simulink library "EmE_MBD_Blockset"  (R2018a)
settings: Solver=ode1  StartTime=0.0  StopTime=Inf  FixedStep=0.001  RelTol=1e-3  EnableMultiTasking=on
PostLoadFcn:
  | , if any(exist('dsrtsu_mdlpostloadfcn', 'file') == [2, 3, 6]), try dsrtsu_mdlpostloadfcn('Execute', bdroot); catch fprintf('Error in PostLoadFcn (dsrtsu_mdlpostloadfcn) for model "%s":\n %s\n', bdroot, lasterr); end, end,
undefined symbols (not defined in the file or in its folder): ENUM_TSC1_CONTROL_PURPOSE_T, gcbh, GLB_SWITCH_T
libraries: simulink x237, $bdroot x115, simulink_need_slupdate x26, MotoHawk_lib x13, simulink_extras x3
(part 6 of 11)

== system EmE_MBD_Blockset/User-Defined Functions/Snoop/CCP_ETC_SS2/Recieve Count ==
  Add : Sum  AccumDataTypeStr=uint8  OutDataTypeStr=uint8
  Constant : Constant  OutDataTypeStr=uint8
  Unit Delay : UnitDelay  SampleTime=-1
  motohawk_probe : MotoHawk_lib/Calibration & Probing Blocks/motohawk_probe  nam='CCP_Snoop_ETCrsp_cnt'  show_more=on  name_source=Use Parameter  read_level=1  view_as=Number  enum_struct={'Disabled', 'Enabled'}  vector_style=Wide Row  use_help_units=off  help=''  units=''  use_header_enum=off  row_header_enum={}  col_header_enum={}  use_min_max=off  min_val=-inf  max_val=inf  use_precision=off  precision=''  gain=1  offset=0  exp=1  use_mototune_group=on  mototune_group='CCP_Snoop'
      settings: SourceProductName=MotoHawk
  wires:
  Unit Delay/1 -> Add/2
  Add/1 -> Unit Delay/1, motohawk_probe/1
  Constant/1 -> Add/1

== system EmE_MBD_Blockset/User-Defined Functions/Snoop/Defaulting/DEFAULT1 ==
  signal : Inport
  reset_delay : Inport  Port=2
  f_defined : Inport  Port=3
  CCP_SIG_DEFAULT : Constant  Value=0
  FGND_RTI_ms : Constant  Value=10
  Switch : Switch  Criteria=u2 ~= 0
  Switch1 : Switch  Criteria=u2 ~= 0
  Turn_off_delay : $bdroot/Discrete/Turn_off_delay
  Unit Delay : UnitDelay  SampleTime=-1
  Signal : Outport
  F_Defined : Outport  Port=2
  wires:
  reset_delay/1 -> Turn_off_delay/2
  Turn_off_delay/1 -> Switch/2, F_Defined/1
  FGND_RTI_ms/1 -> Turn_off_delay/3
  Switch1/1 -> Switch/1, Unit Delay/1
  Unit Delay/1 -> Switch1/3
  Switch/1 -> Signal/1
  signal/1 -> Switch1/1
  CCP_SIG_DEFAULT/1 -> Switch/3
  f_defined/1 -> Turn_off_delay/1, Switch1/2

== system EmE_MBD_Blockset/User-Defined Functions/Snoop/Defaulting/DEFAULT10 ==
  signal : Inport
  reset_delay : Inport  Port=2
  f_defined : Inport  Port=3
  CCP_SIG_DEFAULT : Constant  Value=0
  FGND_RTI_ms : Constant  Value=10
  Switch : Switch  Criteria=u2 ~= 0
  Switch1 : Switch  Criteria=u2 ~= 0
  Turn_off_delay : $bdroot/Discrete/Turn_off_delay
  Unit Delay : UnitDelay  SampleTime=-1
  Signal : Outport
  F_Defined : Outport  Port=2
  wires:
  f_defined/1 -> Switch1/2, Turn_off_delay/1
  CCP_SIG_DEFAULT/1 -> Switch/3
  signal/1 -> Switch1/1
  Switch/1 -> Signal/1
  Unit Delay/1 -> Switch1/3
  Switch1/1 -> Unit Delay/1, Switch/1
  FGND_RTI_ms/1 -> Turn_off_delay/3
  Turn_off_delay/1 -> F_Defined/1, Switch/2
  reset_delay/1 -> Turn_off_delay/2

== system EmE_MBD_Blockset/User-Defined Functions/Snoop/Defaulting/DEFAULT11 ==
  signal : Inport
  reset_delay : Inport  Port=2
  f_defined : Inport  Port=3
  CCP_SIG_DEFAULT : Constant  Value=0
  FGND_RTI_ms : Constant  Value=10
  Switch : Switch  Criteria=u2 ~= 0
  Switch1 : Switch  Criteria=u2 ~= 0
  Turn_off_delay : $bdroot/Discrete/Turn_off_delay
  Unit Delay : UnitDelay  SampleTime=-1
  Signal : Outport
  F_Defined : Outport  Port=2
  wires:
  f_defined/1 -> Switch1/2, Turn_off_delay/1
  CCP_SIG_DEFAULT/1 -> Switch/3
  signal/1 -> Switch1/1
  Switch/1 -> Signal/1
  Unit Delay/1 -> Switch1/3
  Switch1/1 -> Unit Delay/1, Switch/1
  FGND_RTI_ms/1 -> Turn_off_delay/3
  Turn_off_delay/1 -> F_Defined/1, Switch/2
  reset_delay/1 -> Turn_off_delay/2

== system EmE_MBD_Blockset/User-Defined Functions/Snoop/Defaulting/DEFAULT12 ==
  signal : Inport
  reset_delay : Inport  Port=2
  f_defined : Inport  Port=3
  CCP_SIG_DEFAULT : Constant  Value=0
  FGND_RTI_ms : Constant  Value=10
  Switch : Switch  Criteria=u2 ~= 0
  Switch1 : Switch  Criteria=u2 ~= 0
  Turn_off_delay : $bdroot/Discrete/Turn_off_delay
  Unit Delay : UnitDelay  SampleTime=-1
  Signal : Outport
  F_Defined : Outport  Port=2
  wires:
  reset_delay/1 -> Turn_off_delay/2
  Turn_off_delay/1 -> Switch/2, F_Defined/1
  FGND_RTI_ms/1 -> Turn_off_delay/3
  Switch1/1 -> Switch/1, Unit Delay/1
  Unit Delay/1 -> Switch1/3
  Switch/1 -> Signal/1
  signal/1 -> Switch1/1
  CCP_SIG_DEFAULT/1 -> Switch/3
  f_defined/1 -> Turn_off_delay/1, Switch1/2

== system EmE_MBD_Blockset/User-Defined Functions/Snoop/Defaulting/DEFAULT2 ==
  signal : Inport
  reset_delay : Inport  Port=2
  f_defined : Inport  Port=3
  CCP_SIG_DEFAULT : Constant  Value=0
  FGND_RTI_ms : Constant  Value=10
  Switch : Switch  Criteria=u2 ~= 0
  Switch1 : Switch  Criteria=u2 ~= 0
  Turn_off_delay : $bdroot/Discrete/Turn_off_delay
  Unit Delay : UnitDelay  SampleTime=-1
  Signal : Outport
  F_Defined : Outport  Port=2
  wires:
  f_defined/1 -> Switch1/2, Turn_off_delay/1
  CCP_SIG_DEFAULT/1 -> Switch/3
  signal/1 -> Switch1/1
  Switch/1 -> Signal/1
  Unit Delay/1 -> Switch1/3
  Switch1/1 -> Unit Delay/1, Switch/1
  FGND_RTI_ms/1 -> Turn_off_delay/3
  Turn_off_delay/1 -> F_Defined/1, Switch/2
  reset_delay/1 -> Turn_off_delay/2

== system EmE_MBD_Blockset/User-Defined Functions/Snoop/Defaulting/DEFAULT3 ==
  signal : Inport
  reset_delay : Inport  Port=2
  f_defined : Inport  Port=3
  CCP_SIG_DEFAULT : Constant  Value=0
  FGND_RTI_ms : Constant  Value=10
  Switch : Switch  Criteria=u2 ~= 0
  Switch1 : Switch  Criteria=u2 ~= 0
  Turn_off_delay : $bdroot/Discrete/Turn_off_delay
  Unit Delay : UnitDelay  SampleTime=-1
  Signal : Outport
  F_Defined : Outport  Port=2
  wires:
  f_defined/1 -> Switch1/2, Turn_off_delay/1
  CCP_SIG_DEFAULT/1 -> Switch/3
  signal/1 -> Switch1/1
  Switch/1 -> Signal/1
  Unit Delay/1 -> Switch1/3
  Switch1/1 -> Unit Delay/1, Switch/1
  FGND_RTI_ms/1 -> Turn_off_delay/3
  Turn_off_delay/1 -> F_Defined/1, Switch/2
  reset_delay/1 -> Turn_off_delay/2

== system EmE_MBD_Blockset/User-Defined Functions/Snoop/Defaulting/DEFAULT4 ==
  signal : Inport
  reset_delay : Inport  Port=2
  f_defined : Inport  Port=3
  CCP_SIG_DEFAULT : Constant  Value=0
  FGND_RTI_ms : Constant  Value=10
  Switch : Switch  Criteria=u2 ~= 0
  Switch1 : Switch  Criteria=u2 ~= 0
  Turn_off_delay : $bdroot/Discrete/Turn_off_delay
  Unit Delay : UnitDelay  SampleTime=-1
  Signal : Outport
  F_Defined : Outport  Port=2
  wires:
  reset_delay/1 -> Turn_off_delay/2
  Turn_off_delay/1 -> Switch/2, F_Defined/1
  FGND_RTI_ms/1 -> Turn_off_delay/3
  Switch1/1 -> Switch/1, Unit Delay/1
  Unit Delay/1 -> Switch1/3
  Switch/1 -> Signal/1
  signal/1 -> Switch1/1
  CCP_SIG_DEFAULT/1 -> Switch/3
  f_defined/1 -> Turn_off_delay/1, Switch1/2

== system EmE_MBD_Blockset/User-Defined Functions/Snoop/Defaulting/DEFAULT5 ==
  signal : Inport
  reset_delay : Inport  Port=2
  f_defined : Inport  Port=3
  CCP_SIG_DEFAULT : Constant  Value=0
  FGND_RTI_ms : Constant  Value=10
  Switch : Switch  Criteria=u2 ~= 0
  Switch1 : Switch  Criteria=u2 ~= 0
  Turn_off_delay : $bdroot/Discrete/Turn_off_delay
  Unit Delay : UnitDelay  SampleTime=-1
  Signal : Outport
  F_Defined : Outport  Port=2
  wires:
  f_defined/1 -> Switch1/2, Turn_off_delay/1
  CCP_SIG_DEFAULT/1 -> Switch/3
  signal/1 -> Switch1/1
  Switch/1 -> Signal/1
  Unit Delay/1 -> Switch1/3
  Switch1/1 -> Unit Delay/1, Switch/1
  FGND_RTI_ms/1 -> Turn_off_delay/3
  Turn_off_delay/1 -> F_Defined/1, Switch/2
  reset_delay/1 -> Turn_off_delay/2

== system EmE_MBD_Blockset/User-Defined Functions/Snoop/Defaulting/DEFAULT6 ==
  signal : Inport
  reset_delay : Inport  Port=2
  f_defined : Inport  Port=3
  CCP_SIG_DEFAULT : Constant  Value=0
  FGND_RTI_ms : Constant  Value=10
  Switch : Switch  Criteria=u2 ~= 0
  Switch1 : Switch  Criteria=u2 ~= 0
  Turn_off_delay : $bdroot/Discrete/Turn_off_delay
  Unit Delay : UnitDelay  SampleTime=-1
  Signal : Outport
  F_Defined : Outport  Port=2
  wires:
  reset_delay/1 -> Turn_off_delay/2
  Turn_off_delay/1 -> Switch/2, F_Defined/1
  FGND_RTI_ms/1 -> Turn_off_delay/3
  Switch1/1 -> Switch/1, Unit Delay/1
  Unit Delay/1 -> Switch1/3
  Switch/1 -> Signal/1
  signal/1 -> Switch1/1
  CCP_SIG_DEFAULT/1 -> Switch/3
  f_defined/1 -> Turn_off_delay/1, Switch1/2

== system EmE_MBD_Blockset/User-Defined Functions/Snoop/Defaulting/DEFAULT7 ==
  signal : Inport
  reset_delay : Inport  Port=2
  f_defined : Inport  Port=3
  CCP_SIG_DEFAULT : Constant  Value=0
  FGND_RTI_ms : Constant  Value=10
  Switch : Switch  Criteria=u2 ~= 0
  Switch1 : Switch  Criteria=u2 ~= 0
  Turn_off_delay : $bdroot/Discrete/Turn_off_delay
  Unit Delay : UnitDelay  SampleTime=-1
  Signal : Outport
  F_Defined : Outport  Port=2
  wires:
  reset_delay/1 -> Turn_off_delay/2
  Turn_off_delay/1 -> Switch/2, F_Defined/1
  FGND_RTI_ms/1 -> Turn_off_delay/3
  Switch1/1 -> Switch/1, Unit Delay/1
  Unit Delay/1 -> Switch1/3
  Switch/1 -> Signal/1
  signal/1 -> Switch1/1
  CCP_SIG_DEFAULT/1 -> Switch/3
  f_defined/1 -> Turn_off_delay/1, Switch1/2

== system EmE_MBD_Blockset/User-Defined Functions/Snoop/Defaulting/DEFAULT8 ==
  signal : Inport
  reset_delay : Inport  Port=2
  f_defined : Inport  Port=3
  CCP_SIG_DEFAULT : Constant  Value=0
  FGND_RTI_ms : Constant  Value=10
  Switch : Switch  Criteria=u2 ~= 0
  Switch1 : Switch  Criteria=u2 ~= 0
  Turn_off_delay : $bdroot/Discrete/Turn_off_delay
  Unit Delay : UnitDelay  SampleTime=-1
  Signal : Outport
  F_Defined : Outport  Port=2
  wires:
  f_defined/1 -> Switch1/2, Turn_off_delay/1
  CCP_SIG_DEFAULT/1 -> Switch/3
  signal/1 -> Switch1/1
  Switch/1 -> Signal/1
  Unit Delay/1 -> Switch1/3
  Switch1/1 -> Unit Delay/1, Switch/1
  FGND_RTI_ms/1 -> Turn_off_delay/3
  Turn_off_delay/1 -> F_Defined/1, Switch/2
  reset_delay/1 -> Turn_off_delay/2

== system EmE_MBD_Blockset/User-Defined Functions/Snoop/Defaulting/DEFAULT9 ==
  signal : Inport
  reset_delay : Inport  Port=2
  f_defined : Inport  Port=3
  CCP_SIG_DEFAULT : Constant  Value=0
  FGND_RTI_ms : Constant  Value=10
  Switch : Switch  Criteria=u2 ~= 0
  Switch1 : Switch  Criteria=u2 ~= 0
  Turn_off_delay : $bdroot/Discrete/Turn_off_delay
  Unit Delay : UnitDelay  SampleTime=-1
  Signal : Outport
  F_Defined : Outport  Port=2
  wires:
  reset_delay/1 -> Turn_off_delay/2
  Turn_off_delay/1 -> Switch/2, F_Defined/1
  FGND_RTI_ms/1 -> Turn_off_delay/3
  Switch1/1 -> Switch/1, Unit Delay/1
  Unit Delay/1 -> Switch1/3
  Switch/1 -> Signal/1
  signal/1 -> Switch1/1
  CCP_SIG_DEFAULT/1 -> Switch/3
  f_defined/1 -> Turn_off_delay/1, Switch1/2

== system EmE_MBD_Blockset/User-Defined Functions/Snoop/Defaulting/Recieve Count ==
  Add : Sum  AccumDataTypeStr=uint8  OutDataTypeStr=uint8
  Constant : Constant  OutDataTypeStr=uint8
  Unit Delay : UnitDelay  SampleTime=-1
  motohawk_probe : MotoHawk_lib/Calibration & Probing Blocks/motohawk_probe  nam='CCP_Snoop_Default_cnt'  show_more=on  name_source=Use Parameter  read_level=1  view_as=Number  enum_struct={'Disabled', 'Enabled'}  vector_style=Wide Row  use_help_units=off  help=''  units=''  use_header_enum=off  row_header_enum={}  col_header_enum={}  use_min_max=off  min_val=-inf  max_val=inf  use_precision=off  precision=''  gain=1  offset=0  exp=1  use_mototune_group=on  mototune_group='CCP_Snoop'
      settings: SourceProductName=MotoHawk
  wires:
  Constant/1 -> Add/1
  Add/1 -> motohawk_probe/1, Unit Delay/1
  Unit Delay/1 -> Add/2

== system EmE_MBD_Blockset/Controllers/Generic_PID_Governor_3/Calculate_PID_terms/Calculate_I_term/Calculate_integral_term ==
  GPID_dT : Inport
  F_GPID_reset_gov : Inport  Port=2
  GPID_i_sum_error_init : Inport  Port=3
  GPID_control_error : Inport  Port=4
  GPID_Ki : Inport  Port=5
  F_GPID_hold_i_term : Inport  Port=6
  Add : Sum  InputSameDT=on
  If_Then_Else : $bdroot/Signal Routing/If_Then_Else
  Product1 : Product  Inputs=3  InputSameDT=on
  Unit Delay Resettable External IC1 : simulink_need_slupdate/Unit Delay Resettable External IC  tsamp=-1
      settings: SourceProductName=Simulink  SourceProductBaseCode=SL
  GPID_i_term : Outport  OutputWhenDisabled=reset  InitialOutput=0
  wires:
  F_GPID_hold_i_term/1 -> If_Then_Else/1
  If_Then_Else/1 -> Unit Delay Resettable External IC1/1, GPID_i_term/1
  F_GPID_reset_gov/1 -> Unit Delay Resettable External IC1/2
  GPID_i_sum_error_init/1 -> Unit Delay Resettable External IC1/3
  Unit Delay Resettable External IC1/1 -> If_Then_Else/2, Add/1
  Product1/1 -> Add/2
  Add/1 -> If_Then_Else/3
  GPID_dT/1 -> Product1/3
  GPID_control_error/1 -> Product1/2
  GPID_Ki/1 -> Product1/1

== system EmE_MBD_Blockset/Controllers/Generic_PID_Governor_3/Calculate_PID_terms/Calculate_I_term/Initialize_integral_term ==
  GPID_dT : Inport
  GPID_feed_forward : Inport  Port=2
  GPID_p_term : Inport  Port=3
  GPID_actual_system_output : Inport  Port=4
  GPID_control_error : Inport  Port=5
  GPID_Ki : Inport  Port=6
  Enable : EnablePort
      settings: AttributesFormatString=States when enabling: %<StatesWhenEnabling>
  Product : Product  Inputs=3  InputSameDT=on
  Subtract : Sum  Inputs=+-  InputSameDT=on
  Subtract1 : Sum  Inputs=+-  InputSameDT=on
  Subtract2 : Sum  Inputs=+-  InputSameDT=on
  GPID_i_sum_error_init : Outport  InitialOutput=0
      settings: AttributesFormatString=IC: %<InitialOutput>\nDisabled value: %<OutputWhenDisabled>
  wires:
  Subtract2/1 -> GPID_i_sum_error_init/1
  GPID_actual_system_output/1 -> Subtract/1
  GPID_feed_forward/1 -> Subtract/2
  Subtract/1 -> Subtract1/1
  GPID_p_term/1 -> Subtract1/2
  Subtract1/1 -> Subtract2/1
  Product/1 -> Subtract2/2
  GPID_Ki/1 -> Product/1
  GPID_dT/1 -> Product/2
  GPID_control_error/1 -> Product/3

== system EmE_MBD_Blockset/Controllers/Generic_PID_Governor_3/Calculate_PID_terms/Calculate_I_term/Prevent_integral_term_windup ==
  GPID_Ki : Inport
  GPID_control_error : Inport  Port=2
  GPID_actual_system_output : Inport  Port=3
  F_GPID_reset_gov : Inport  Port=4
  GPID_output_unlim_prev : Inport  Port=5
  F_GPID_aw_cond_integration : Inport  Port=6
  GPID_aw_hysteresis : Inport  Port=7
  F_GPID_aw_hold_i_term : Inport  Port=8
  GPID_i_term_prev : Inport  Port=9
  Compare To Zero : simulink/Logic and Bit Operations/Compare To Zero  relop=>  OutDataTypeStr=boolean
  Compare To Zero1 : simulink/Logic and Bit Operations/Compare To Zero  relop=>=  OutDataTypeStr=boolean
  Constant : Constant  Value=0
  If_Then_Else{,1..3} (4 alike) : $bdroot/Signal Routing/If_Then_Else
  Logical Operator1 : $bdroot/Logic and Bit Operations/Logical Operator  Operator=AND  Inputs=2
  Logical Operator2 : $bdroot/Logic and Bit Operations/Logical Operator  Operator=OR  Inputs=2
  Product : Product  Inputs=3  InputSameDT=on
  Relational Operator1 : $bdroot/Logic and Bit Operations/Relational Operator  func=>
  Relational Operator2 : $bdroot/Logic and Bit Operations/Relational Operator  func=>
  Subtract : Sum  Inputs=+-  InputSameDT=on
  Subtract1 : Sum  Inputs=+-  InputSameDT=on
  F_GPID_hold_i_term : Outport  OutputWhenDisabled=reset  InitialOutput=false
  wires:
  Constant/1 -> If_Then_Else/2
  GPID_Ki/1 -> Product/1
  GPID_control_error/1 -> Product/2
  F_GPID_aw_cond_integration/1 -> If_Then_Else1/1
  F_GPID_reset_gov/1 -> If_Then_Else2/1, If_Then_Else/1
  GPID_i_term_prev/1 -> Compare To Zero1/1, If_Then_Else/3
  If_Then_Else/1 -> If_Then_Else1/2
  GPID_actual_system_output/1 -> Subtract/2, Subtract1/1, If_Then_Else2/2
  GPID_output_unlim_prev/1 -> If_Then_Else2/3
  If_Then_Else2/1 -> Subtract1/2, Subtract/1, If_Then_Else1/3
  If_Then_Else1/1 -> Product/3
  Product/1 -> Compare To Zero/1
  Compare To Zero1/1 -> If_Then_Else3/1
  Logical Operator2/1 -> F_GPID_hold_i_term/1
  Subtract/1 -> Relational Operator1/1
  Subtract1/1 -> Relational Operator2/1
  GPID_aw_hysteresis/1 -> Relational Operator2/2, Relational Operator1/2
  Relational Operator1/1 -> If_Then_Else3/2
  Relational Operator2/1 -> If_Then_Else3/3
  Compare To Zero/1 -> Logical Operator1/1
  If_Then_Else3/1 -> Logical Operator1/2
  F_GPID_aw_hold_i_term/1 -> Logical Operator2/2
  Logical Operator1/1 -> Logical Operator2/1

== system EmE_MBD_Blockset/Controllers/Generic_PID_Governor_4/Calculate_PID_terms/Calculate_I_term/Calculate_integral_term ==
  GPID_dT : Inport
  F_GPID_reset_gov : Inport  Port=2
  GPID_i_sum_error_init : Inport  Port=3
  GPID_control_error : Inport  Port=4
  GPID_Ki : Inport  Port=5
  GPID_output_delta : Inport  Port=6
  F_GPID_hold_i_term : Inport  Port=7
  Add : Sum  InputSameDT=on
  Add1 : Sum  InputSameDT=on
  CPV : Constant  Value=0
  GPID_AW_USE_FEEDBACK_DELTA_CPV : Constant  Value=false
  If_Then_Else : $bdroot/Signal Routing/If_Then_Else
  If_Then_Else1 : $bdroot/Signal Routing/If_Then_Else
  Product : Product  InputSameDT=on
  Product1 : Product  InputSameDT=on
  Unit Delay Resettable External IC1 : simulink_need_slupdate/Unit Delay Resettable External IC  tsamp=-1
      settings: SourceProductName=Simulink  SourceProductBaseCode=SL
  GPID_i_term : Outport  OutputWhenDisabled=reset  InitialOutput=0
  wires:
  F_GPID_hold_i_term/1 -> If_Then_Else/1
  If_Then_Else/1 -> Unit Delay Resettable External IC1/1, GPID_i_term/1
  F_GPID_reset_gov/1 -> Unit Delay Resettable External IC1/2
  GPID_i_sum_error_init/1 -> Unit Delay Resettable External IC1/3
  GPID_dT/1 -> Product1/2
  GPID_Ki/1 -> Product/1
  GPID_control_error/1 -> Product/2
  Unit Delay Resettable External IC1/1 -> If_Then_Else/2, Add/1
  Product1/1 -> Add/2
  Add/1 -> If_Then_Else/3
  Product/1 -> Add1/1
  GPID_output_delta/1 -> If_Then_Else1/2
  GPID_AW_USE_FEEDBACK_DELTA_CPV/1 -> If_Then_Else1/1
  Add1/1 -> Product1/1
  CPV/1 -> If_Then_Else1/3
  If_Then_Else1/1 -> Add1/2

== system EmE_MBD_Blockset/Controllers/Generic_PID_Governor_4/Calculate_PID_terms/Calculate_I_term/Initialize_integral_term ==
  GPID_dT : Inport
  GPID_feed_forward : Inport  Port=2
  GPID_p_term : Inport  Port=3
  GPID_actual_system_output : Inport  Port=4
  GPID_control_error : Inport  Port=5
  GPID_Ki : Inport  Port=6
  Enable : EnablePort
      settings: AttributesFormatString=States when enabling: %<StatesWhenEnabling>
  Product : Product  Inputs=3  InputSameDT=on
  Subtract : Sum  Inputs=+-  InputSameDT=on
  Subtract1 : Sum  Inputs=+-  InputSameDT=on
  Subtract2 : Sum  Inputs=+-  InputSameDT=on
  GPID_i_sum_error_init : Outport  InitialOutput=0
      settings: AttributesFormatString=IC: %<InitialOutput>\nDisabled value: %<OutputWhenDisabled>
  wires:
  Subtract2/1 -> GPID_i_sum_error_init/1
  GPID_actual_system_output/1 -> Subtract/1
  GPID_feed_forward/1 -> Subtract/2
  Subtract/1 -> Subtract1/1
  GPID_p_term/1 -> Subtract1/2
  Subtract1/1 -> Subtract2/1
  Product/1 -> Subtract2/2
  GPID_Ki/1 -> Product/1
  GPID_dT/1 -> Product/2
  GPID_control_error/1 -> Product/3

== system EmE_MBD_Blockset/Controllers/Generic_PID_Governor_4/Calculate_PID_terms/Calculate_I_term/Prevent_integral_term_windup ==
  GPID_Ki : Inport
  GPID_control_error : Inport  Port=2
  GPID_actual_system_output : Inport  Port=3
  F_GPID_reset_gov : Inport  Port=4
  GPID_output_unlim_prev : Inport  Port=5
  F_GPID_aw_cond_integration : Inport  Port=6
  GPID_aw_hysteresis : Inport  Port=7
  F_GPID_aw_hold_i_term : Inport  Port=8
  GPID_i_term_prev : Inport  Port=9
  Compare To Zero : simulink/Logic and Bit Operations/Compare To Zero  relop=>  OutDataTypeStr=boolean
  Compare To Zero1 : simulink/Logic and Bit Operations/Compare To Zero  relop=>=  OutDataTypeStr=boolean
  Constant : Constant  Value=0
  If_Then_Else{,1..3} (4 alike) : $bdroot/Signal Routing/If_Then_Else
  Logical Operator1 : $bdroot/Logic and Bit Operations/Logical Operator  Operator=AND  Inputs=2
  Logical Operator2 : $bdroot/Logic and Bit Operations/Logical Operator  Operator=OR  Inputs=2
  Product : Product  Inputs=3  InputSameDT=on
  Relational Operator1 : $bdroot/Logic and Bit Operations/Relational Operator  func=>
  Relational Operator2 : $bdroot/Logic and Bit Operations/Relational Operator  func=>
  Subtract : Sum  Inputs=+-  InputSameDT=on
  Subtract1 : Sum  Inputs=+-  InputSameDT=on
  F_GPID_hold_i_term : Outport  OutputWhenDisabled=reset  InitialOutput=false
  wires:
  Constant/1 -> If_Then_Else/2
  GPID_Ki/1 -> Product/1
  GPID_control_error/1 -> Product/2
  F_GPID_aw_cond_integration/1 -> If_Then_Else1/1
  F_GPID_reset_gov/1 -> If_Then_Else2/1, If_Then_Else/1
  GPID_i_term_prev/1 -> Compare To Zero1/1, If_Then_Else/3
  If_Then_Else/1 -> If_Then_Else1/2
  GPID_actual_system_output/1 -> Subtract/2, Subtract1/1, If_Then_Else2/2
  GPID_output_unlim_prev/1 -> If_Then_Else2/3
  If_Then_Else2/1 -> Subtract1/2, Subtract/1, If_Then_Else1/3
  If_Then_Else1/1 -> Product/3
  Product/1 -> Compare To Zero/1
  Compare To Zero1/1 -> If_Then_Else3/1
  Logical Operator2/1 -> F_GPID_hold_i_term/1
  Subtract/1 -> Relational Operator1/1
  Subtract1/1 -> Relational Operator2/1
  GPID_aw_hysteresis/1 -> Relational Operator2/2, Relational Operator1/2
  Relational Operator1/1 -> If_Then_Else3/2
  Relational Operator2/1 -> If_Then_Else3/3
  Compare To Zero/1 -> Logical Operator1/1
  If_Then_Else3/1 -> Logical Operator1/2
  F_GPID_aw_hold_i_term/1 -> Logical Operator2/2
  Logical Operator1/1 -> Logical Operator2/1

== system EmE_MBD_Blockset/User-Defined Functions/Snoop/CCP_ETC_SS1/CCP Signal Data Configuration/SignalDef1 ==
  Address : Constant  Value=hex2dec('400076EC')  OutDataTypeStr=uint32
  Bus Creator4 : BusCreator  Inputs=3
  Conversion : Constant  Value="[1  1  0]"  OutDataTypeStr=double
  DataType : Constant  Value=bin2dec('0000')  OutDataTypeStr=uint8
  Signal_Info : Outport
  wires:
  Address/1 -> Bus Creator4/1  "Signal_Address"
  DataType/1 -> Bus Creator4/2  "Signal_Type"
  Conversion/1 -> Bus Creator4/3  "Signal_Conversion"
  Bus Creator4/1 -> Signal_Info/1

== system EmE_MBD_Blockset/User-Defined Functions/Snoop/CCP_ETC_SS1/CCP Signal Data Configuration/SignalDef10 ==
  Address : Constant  Value=hex2dec('00501F12')  OutDataTypeStr=uint32
  Bus Creator4 : BusCreator  Inputs=3
  Conversion : Constant  Value="[1  10   0]"  OutDataTypeStr=double
  DataType : Constant  Value=bin2dec('0011')  OutDataTypeStr=uint8
  Signal_Info : Outport
  wires:
  Bus Creator4/1 -> Signal_Info/1
  Conversion/1 -> Bus Creator4/3  "Signal_Conversion"
  DataType/1 -> Bus Creator4/2  "Signal_Type"
  Address/1 -> Bus Creator4/1  "Signal_Address"

== system EmE_MBD_Blockset/User-Defined Functions/Snoop/CCP_ETC_SS1/CCP Signal Data Configuration/SignalDef11 ==
  Address : Constant  Value=hex2dec('4000C33C')  OutDataTypeStr=uint32
  Bus Creator4 : BusCreator  Inputs=3
  Conversion : Constant  Value="[1  10   0]"  OutDataTypeStr=double
  DataType : Constant  Value=bin2dec('1011')  OutDataTypeStr=uint8
  Signal_Info : Outport
  wires:
  Bus Creator4/1 -> Signal_Info/1
  Conversion/1 -> Bus Creator4/3  "Signal_Conversion"
  DataType/1 -> Bus Creator4/2  "Signal_Type"
  Address/1 -> Bus Creator4/1  "Signal_Address"

== system EmE_MBD_Blockset/User-Defined Functions/Snoop/CCP_ETC_SS1/CCP Signal Data Configuration/SignalDef12 ==
  Address : Constant  Value=hex2dec('40007564')  OutDataTypeStr=uint32
  Bus Creator4 : BusCreator  Inputs=3
  Conversion : Constant  Value="[1  1  0]"  OutDataTypeStr=double
  DataType : Constant  Value=bin2dec('0000')  OutDataTypeStr=uint8
  Signal_Info : Outport
  wires:
  Bus Creator4/1 -> Signal_Info/1
  Conversion/1 -> Bus Creator4/3  "Signal_Conversion"
  DataType/1 -> Bus Creator4/2  "Signal_Type"
  Address/1 -> Bus Creator4/1  "Signal_Address"

== system EmE_MBD_Blockset/User-Defined Functions/Snoop/CCP_ETC_SS1/CCP Signal Data Configuration/SignalDef2 ==
  Address : Constant  Value=hex2dec('40007D66')  OutDataTypeStr=uint32
  Bus Creator4 : BusCreator  Inputs=3
  Conversion : Constant  Value="[1  1  0]"  OutDataTypeStr=double
  DataType : Constant  Value=bin2dec('0011')  OutDataTypeStr=uint8
  Signal_Info : Outport
  wires:
  Bus Creator4/1 -> Signal_Info/1
  Conversion/1 -> Bus Creator4/3  "Signal_Conversion"
  DataType/1 -> Bus Creator4/2  "Signal_Type"
  Address/1 -> Bus Creator4/1  "Signal_Address"

== system EmE_MBD_Blockset/User-Defined Functions/Snoop/CCP_ETC_SS1/CCP Signal Data Configuration/SignalDef3 ==
  Address : Constant  Value=hex2dec('4000C33A')  OutDataTypeStr=uint32
  Bus Creator4 : BusCreator  Inputs=3
  Conversion : Constant  Value="[1  10   0]"  OutDataTypeStr=double
  DataType : Constant  Value=bin2dec('0011')  OutDataTypeStr=uint8
  Signal_Info : Outport
  wires:
  Address/1 -> Bus Creator4/1  "Signal_Address"
  DataType/1 -> Bus Creator4/2  "Signal_Type"
  Conversion/1 -> Bus Creator4/3  "Signal_Conversion"
  Bus Creator4/1 -> Signal_Info/1

== system EmE_MBD_Blockset/User-Defined Functions/Snoop/CCP_ETC_SS1/CCP Signal Data Configuration/SignalDef4 ==
  Address : Constant  Value=hex2dec('4000BF4A')  OutDataTypeStr=uint32
  Bus Creator4 : BusCreator  Inputs=3
  Conversion : Constant  Value="[1  40   0]"  OutDataTypeStr=double
  DataType : Constant  Value=bin2dec('0011')  OutDataTypeStr=uint8
  Signal_Info : Outport
  wires:
  Bus Creator4/1 -> Signal_Info/1
  Conversion/1 -> Bus Creator4/3  "Signal_Conversion"
  DataType/1 -> Bus Creator4/2  "Signal_Type"
  Address/1 -> Bus Creator4/1  "Signal_Address"

== system EmE_MBD_Blockset/User-Defined Functions/Snoop/CCP_ETC_SS1/CCP Signal Data Configuration/SignalDef5 ==
  Address : Constant  Value=hex2dec('4000768C')  OutDataTypeStr=uint32
  Bus Creator4 : BusCreator  Inputs=3
  Conversion : Constant  Value="[1  1  0]"  OutDataTypeStr=double
  DataType : Constant  Value=bin2dec('0000')  OutDataTypeStr=uint8
  Signal_Info : Outport
  wires:
  Bus Creator4/1 -> Signal_Info/1
  Conversion/1 -> Bus Creator4/3  "Signal_Conversion"
  DataType/1 -> Bus Creator4/2  "Signal_Type"
  Address/1 -> Bus Creator4/1  "Signal_Address"

== system EmE_MBD_Blockset/User-Defined Functions/Snoop/CCP_ETC_SS1/CCP Signal Data Configuration/SignalDef6 ==
  Address : Constant  Value=hex2dec('40007530')  OutDataTypeStr=uint32
  Bus Creator4 : BusCreator  Inputs=3
  Conversion : Constant  Value="[1  1  0]"  OutDataTypeStr=double
  DataType : Constant  Value=bin2dec('0000')  OutDataTypeStr=uint8
  Signal_Info : Outport
  wires:
  Bus Creator4/1 -> Signal_Info/1
  Conversion/1 -> Bus Creator4/3  "Signal_Conversion"
  DataType/1 -> Bus Creator4/2  "Signal_Type"
  Address/1 -> Bus Creator4/1  "Signal_Address"

== system EmE_MBD_Blockset/User-Defined Functions/Snoop/CCP_ETC_SS1/CCP Signal Data Configuration/SignalDef7 ==
  Address : Constant  Value=hex2dec('4000750C')  OutDataTypeStr=uint32
  Bus Creator4 : BusCreator  Inputs=3
  Conversion : Constant  Value="[1  1  0]"  OutDataTypeStr=double
  DataType : Constant  Value=bin2dec('0000')  OutDataTypeStr=uint8
  Signal_Info : Outport
  wires:
  Bus Creator4/1 -> Signal_Info/1
  Conversion/1 -> Bus Creator4/3  "Signal_Conversion"
  DataType/1 -> Bus Creator4/2  "Signal_Type"
  Address/1 -> Bus Creator4/1  "Signal_Address"

== system EmE_MBD_Blockset/User-Defined Functions/Snoop/CCP_ETC_SS1/CCP Signal Data Configuration/SignalDef8 ==
  Address : Constant  Value=hex2dec('40006210')  OutDataTypeStr=uint32
  Bus Creator4 : BusCreator  Inputs=3
  Conversion : Constant  Value="[1  1  0]"  OutDataTypeStr=double
  DataType : Constant  Value=bin2dec('0111')  OutDataTypeStr=uint8
  Signal_Info : Outport
  wires:
  Bus Creator4/1 -> Signal_Info/1
  Conversion/1 -> Bus Creator4/3  "Signal_Conversion"
  DataType/1 -> Bus Creator4/2  "Signal_Type"
  Address/1 -> Bus Creator4/1  "Signal_Address"

== system EmE_MBD_Blockset/User-Defined Functions/Snoop/CCP_ETC_SS1/CCP Signal Data Configuration/SignalDef9 ==
  Address : Constant  Value=hex2dec('4000C324')  OutDataTypeStr=uint32
  Bus Creator4 : BusCreator  Inputs=3
  Conversion : Constant  Value="[1  1  0]"  OutDataTypeStr=double
  DataType : Constant  Value=bin2dec('0001')  OutDataTypeStr=uint8
  Signal_Info : Outport
  wires:
  Bus Creator4/1 -> Signal_Info/1
  Conversion/1 -> Bus Creator4/3  "Signal_Conversion"
  DataType/1 -> Bus Creator4/2  "Signal_Type"
  Address/1 -> Bus Creator4/1  "Signal_Address"

== system EmE_MBD_Blockset/User-Defined Functions/Snoop/CCP_ETC_SS1/Process CCP Commands/Process GET_DAQ ==
  Byte1 : Inport
  Byte2 : Inport  Port=2
  Byte3 : Inport  Port=3
  Byte4 : Inport  Port=4
  Byte5 : Inport  Port=5
  Byte6 : Inport  Port=6
  Byte7 : Inport  Port=7
  Byte8 : Inport  Port=8
  Add : Sum  Inputs=++++
  Bus Creator : BusCreator  Inputs=4
  Data Type Conversion{,1..3} (4 alike) : DataTypeConversion  OutDataTypeStr=uint32
  GET_DAQ : Constant  Value=hex2dec('14')  OutDataTypeStr=uint8
  Relational Operator1 : RelationalOperator  Operator===  OutDataTypeStr=boolean  RndMeth=Nearest
  Shift Arithmetic1 : ArithShift
  Shift Arithmetic2 : ArithShift
  Shift Arithmetic3 : ArithShift
  Switch2 : Switch  Criteria=u2 ~= 0
  Terminator : Terminator
  Unit Delay2 : UnitDelay  SampleTime=-1
  CMD_info : Outport
  wires:
  Unit Delay2/1 -> Switch2/3
  Relational Operator1/1 -> Switch2/2
  Switch2/1 -> Unit Delay2/1, CMD_info/1
  Bus Creator/1 -> Switch2/1  "CMD_Info"
  GET_DAQ/1 -> Relational Operator1/1
  Data Type Conversion3/1 -> Add/4
  Data Type Conversion2/1 -> Shift Arithmetic2/1
  Data Type Conversion1/1 -> Shift Arithmetic1/1
  Data Type Conversion/1 -> Shift Arithmetic3/1
  Add/1 -> Bus Creator/4  "DTO_CAN_ID"
  Byte8/1 -> Data Type Conversion3/1
  Shift Arithmetic2/1 -> Add/3
  Shift Arithmetic1/1 -> Add/2
  Shift Arithmetic3/1 -> Add/1
  Byte7/1 -> Data Type Conversion2/1
  Byte6/1 -> Data Type Conversion1/1
  Byte5/1 -> Data Type Conversion/1
  Byte4/1 -> Terminator/1
  Byte3/1 -> Bus Creator/3  "DAQ_Number"
  Byte2/1 -> Bus Creator/2  "CTR"
  Byte1/1 -> Relational Operator1/2, Bus Creator/1  "Cmd_Code"

== system EmE_MBD_Blockset/User-Defined Functions/Snoop/CCP_ETC_SS1/Process CCP Commands/Process SET_DAQ ==
  Byte1 : Inport
  Byte2 : Inport  Port=2
  Byte3 : Inport  Port=3
  Byte4 : Inport  Port=4
  Byte5 : Inport  Port=5
  Bus Creator : BusCreator  Inputs=5
  Relational Operator3 : RelationalOperator  Operator===  OutDataTypeStr=boolean  RndMeth=Nearest
  SET_DAQ : Constant  Value=hex2dec('15')  OutDataTypeStr=uint8
  Switch2 : Switch  Criteria=u2 ~= 0
  Unit Delay2 : UnitDelay  SampleTime=-1
  CMD_info : Outport
  wires:
  Relational Operator3/1 -> Switch2/2
  SET_DAQ/1 -> Relational Operator3/1
  Bus Creator/1 -> Switch2/1  "CMD_Info"
  Unit Delay2/1 -> Switch2/3
  Switch2/1 -> CMD_info/1, Unit Delay2/1
  Byte5/1 -> Bus Creator/5  "Element_Number"
  Byte4/1 -> Bus Creator/4  "ODT_Number"
  Byte3/1 -> Bus Creator/3  "DAQ_Number"
  Byte2/1 -> Bus Creator/2  "CTR"
  Byte1/1 -> Relational Operator3/2, Bus Creator/1  "Cmd_Code"

== system EmE_MBD_Blockset/User-Defined Functions/Snoop/CCP_ETC_SS1/Process CCP Commands/Process START_STOP ==
  note: Stop command for single DAQ
  Byte1 : Inport
  Byte3 : Inport  Port=2
  Byte4 : Inport  Port=3
  DISCONNECT : Constant  Value=hex2dec('7')  OutDataTypeStr=uint8
  End of Session : simulink/Logic and Bit Operations/Compare To Constant  relop===  const=1  OutDataTypeStr=uint8
  Logical Operator : Logic  AllPortsSameDT=off  OutDataTypeStr=boolean
  Logical Operator1 : Logic  AllPortsSameDT=off  OutDataTypeStr=boolean
  Logical Operator2 : Logic  AllPortsSameDT=off  OutDataTypeStr=boolean
  Logical Operator3 : Logic  Operator=OR  AllPortsSameDT=off  OutDataTypeStr=boolean
  Relational Operator1 : RelationalOperator  Operator===  OutDataTypeStr=boolean  RndMeth=Nearest
  Relational Operator2 : RelationalOperator  Operator===  OutDataTypeStr=boolean  RndMeth=Nearest
  Relational Operator3 : RelationalOperator  Operator===  OutDataTypeStr=boolean  RndMeth=Nearest
  Reset ALL : Constant  Value=250  OutDataTypeStr=uint8
  Reset None : Constant  Value=255  OutDataTypeStr=uint8
  START_STOP : Constant  Value=hex2dec('6')  OutDataTypeStr=uint8
  START_STOP_ALL : Constant  Value=hex2dec('8')  OutDataTypeStr=uint8
  Stop All : simulink/Logic and Bit Operations/Compare To Constant  relop===  const=0  OutDataTypeStr=uint8
  Stop DAQ : simulink/Logic and Bit Operations/Compare To Constant  relop===  const=0  OutDataTypeStr=uint8
  Switch1 : Switch  Criteria=u2 ~= 0
  Switch2 : Switch  Criteria=u2 ~= 0
  STRT_STP : Outport
  wires:
  Switch1/1 -> Switch2/3
  Byte1/1 -> Relational Operator1/2, Relational Operator2/2, Relational Operator3/2  "Cmd_Code"
  Byte3/1 -> [B3], Stop DAQ/1
  START_STOP_ALL/1 -> Relational Operator1/1
  Switch2/1 -> STRT_STP/1  "ResetDAQ"
  Byte4/1 -> Switch1/1
  [B3] -> Stop All/1
  Relational Operator1/1 -> Logical Operator/1
  Stop All/1 -> Logical Operator/2
  DISCONNECT/1 -> Relational Operator2/1
  [B3] -> End of Session/1
  End of Session/1 -> Logical Operator1/2
  Relational Operator2/1 -> Logical Operator1/1
  START_STOP/1 -> Relational Operator3/1
  Stop DAQ/1 -> Logical Operator2/2
  Relational Operator3/1 -> Logical Operator2/1
  Logical Operator/1 -> Logical Operator3/1
  Reset ALL/1 -> Switch2/1
  Logical Operator1/1 -> Logical Operator3/2
  Logical Operator3/1 -> Switch2/2
  Logical Operator2/1 -> Switch1/2
  Reset None/1 -> Switch1/3

== system EmE_MBD_Blockset/User-Defined Functions/Snoop/CCP_ETC_SS1/Process CCP Commands/Process WRITE_DAQ ==
  Byte1 : Inport
  Byte2 : Inport  Port=2
  Byte3 : Inport  Port=3
  Byte4 : Inport  Port=4
  Byte5 : Inport  Port=5
  Byte6 : Inport  Port=6
  Byte7 : Inport  Port=7
  Byte8 : Inport  Port=8
  Add : Sum  Inputs=++++  OutDataTypeStr=uint32
  Bus Creator : BusCreator  Inputs=5
  Bus Creator1 : BusCreator  Inputs=5
  Bus Selector : BusSelector  OutputSignals=Cmd_Code,CTR,Element_Size,Address_Extension
  Data Type Conversion{,1..3} (4 alike) : DataTypeConversion  OutDataTypeStr=uint32
  MAX UINT32 : Constant  Value=hex2dec('FFFFFFFF')  OutDataTypeStr=uint32
  Relational Operator3 : RelationalOperator  Operator===  OutDataTypeStr=boolean  RndMeth=Nearest
  Shift Arithmetic1 : ArithShift
  Shift Arithmetic2 : ArithShift
  Shift Arithmetic3 : ArithShift
  Switch2 : Switch  Criteria=u2 ~= 0
  Unit Delay : UnitDelay  SampleTime=-1
  WRITE_DAQ : Constant  Value=hex2dec('16')  OutDataTypeStr=uint8
  CMD_info : Outport
  wires:
  Unit Delay/1 -> Bus Selector/1
  MAX UINT32/1 -> Bus Creator1/5  "Memory_Address"
  Bus Selector/4 -> Bus Creator1/4  "<Address_Extension>"
  Bus Selector/3 -> Bus Creator1/3  "<Element_Size>"
  Bus Selector/2 -> Bus Creator1/2  "<CTR>"
  Bus Selector/1 -> Bus Creator1/1  "<Cmd_Code>"
  Bus Creator1/1 -> Switch2/3
  Relational Operator3/1 -> Switch2/2
  Bus Creator/1 -> Switch2/1  "CMD_Info"
  WRITE_DAQ/1 -> Relational Operator3/1
  Switch2/1 -> Unit Delay/1, CMD_info/1
  Add/1 -> Bus Creator/5  "Memory_Address"
  Byte8/1 -> Data Type Conversion3/1
  Byte7/1 -> Data Type Conversion2/1
  Byte6/1 -> Data Type Conversion1/1
  Byte5/1 -> Data Type Conversion/1
  Data Type Conversion3/1 -> Add/4
  Data Type Conversion2/1 -> Shift Arithmetic2/1
  Data Type Conversion1/1 -> Shift Arithmetic1/1
  Data Type Conversion/1 -> Shift Arithmetic3/1
  Shift Arithmetic2/1 -> Add/3
  Shift Arithmetic1/1 -> Add/2
  Shift Arithmetic3/1 -> Add/1
  Byte4/1 -> Bus Creator/4  "Address_Extension"
  Byte3/1 -> Bus Creator/3  "Element_Size"
  Byte1/1 -> Relational Operator3/2, Bus Creator/1  "Cmd_Code"
  Byte2/1 -> Bus Creator/2  "CTR"

== system EmE_MBD_Blockset/User-Defined Functions/Snoop/CCP_ETC_SS1/Signal Data Pairing/Reset Override ==
  STRT_STP : Inport
  Switch : Switch  Criteria=u2 ~= 0
  motohawk_calibration : MotoHawk_lib/Calibration & Probing Blocks/motohawk_calibration  nam='CCP_SNOOP_RESET_ENABLE'  val=0  storage=Calibration  show_more=on  name_source=Use Parameter  data_type=boolean  read_level=1  write_level=1  ovr_cals=on  view_as=Number  enum_struct={'Disabled', 'Enabled'}  vector_style=Wide Row  use_help_units=off  help=''  units=''  use_header_enum=off  row_header_enum={}  col_header_enum={}  use_min_max=off  min_val=-inf  max_val=inf  use_precision=off  precision=''  gain=1  offset=0  exp=1  use_mototune_group=on  mototune_group='CCP_Snoop'  data_stores=motohawk_sfun_calibration_data_stores
      settings: SourceProductName=MotoHawk
  motohawk_calibration1 : MotoHawk_lib/Calibration & Probing Blocks/motohawk_calibration  nam='CCP_SNOOP_RESET'  val=0  storage=Calibration  show_more=on  name_source=Use Parameter  data_type=uint8  read_level=1  write_level=1  ovr_cals=on  view_as=Number  enum_struct={'Disabled', 'Enabled'}  vector_style=Wide Row  use_help_units=off  help=''  units=''  use_header_enum=off  row_header_enum={}  col_header_enum={}  use_min_max=off  min_val=-inf  max_val=inf  use_precision=off  precision=''  gain=1  offset=0  exp=1  use_mototune_group=on  mototune_group='CCP_Snoop'  data_stores=motohawk_sfun_calibration_data_stores
      settings: SourceProductName=MotoHawk
  motohawk_probe : MotoHawk_lib/Calibration & Probing Blocks/motohawk_probe  nam='CCP_Snoop_ResetDAQ'  show_more=on  name_source=Use Parameter  read_level=1  view_as=Number  enum_struct={'Disabled', 'Enabled'}  vector_style=Wide Row  use_help_units=off  help=''  units=''  use_header_enum=off  row_header_enum={}  col_header_enum={}  use_min_max=off  min_val=-inf  max_val=inf  use_precision=off  precision=''  gain=1  offset=0  exp=1  use_mototune_group=on  mototune_group='CCP_Snoop'
      settings: SourceProductName=MotoHawk
  Connect_reset : Outport
  wires:
  motohawk_calibration1/1 -> Switch/1
  motohawk_calibration/1 -> Switch/2
  Switch/1 -> Connect_reset/1, motohawk_probe/1
  STRT_STP/1 -> Switch/3

== system EmE_MBD_Blockset/User-Defined Functions/Snoop/CCP_ETC_SS1/Signal Data Pairing/Update Signal1 ==
  note: Memory address currently being configured
  note: Configured signal information
  PID : Inport
  Offset : Inport  Port=2
  ResetDAQ : Inport  Port=3
  Memory_Address : Inport  Port=4
  Signal_Info : Inport  Port=5
  Bus Creator : BusCreator  Inputs=6
  Bus Selector1 : BusSelector  OutputSignals=Signal_Address,Signal_Type,Signal_Conversion
  Detect Rise Positive : simulink/Logic and Bit Operations/Detect Rise Positive  vinit=0  InputProcessing=Inherited  OutDataTypeStr=uint8
  Latch w Update : Subsystem
  Latch w Update1 : Subsystem
  RS Flop-Flop Rp : Subsystem
      mask help: RS flip-flop with priority on R
  Relational Operator2 : RelationalOperator  Operator===  OutDataTypeStr=boolean  RndMeth=Nearest
  Reset Logic : Subsystem
  Terminator : Terminator
  Signal_Data_Updated : Outport
  wires:
  RS Flop-Flop Rp/2(!Q) -> Terminator/1
  RS Flop-Flop Rp/1(Q) -> Bus Creator/3  "F_Defined"
  Detect Rise Positive/1 -> Latch w Update1/1(f_update), Latch w Update/1(f_update)
  Bus Selector1/3 -> Bus Creator/6  "<Signal_Conversion>"
  PID/1 -> Latch w Update/2(In)
  Offset/1 -> Latch w Update1/2(In)
  Latch w Update1/1(Latched) -> Bus Creator/2  "Offset"
  Latch w Update/1(Latched) -> Bus Creator/1, [PID]  "PID"
  Bus Creator/1 -> Signal_Data_Updated/1
  Signal_Info/1 -> Bus Selector1/1
  Memory_Address/1 -> Relational Operator2/1
  Relational Operator2/1 -> RS Flop-Flop Rp/2(S), Detect Rise Positive/1  "F_Signal_Defined"
  Bus Selector1/2 -> Bus Creator/5  "<Signal_Type>"
  Bus Selector1/1 -> Bus Creator/4, Relational Operator2/2  "<Signal_Address>"
  Reset Logic/1(Reset) -> RS Flop-Flop Rp/1(Rp)
  ResetDAQ/1 -> Reset Logic/2(ResetDAQ)
  [PID] -> Reset Logic/1(CurrentPID)

== system EmE_MBD_Blockset/User-Defined Functions/Snoop/CCP_ETC_SS1/Signal Data Pairing/Update Signal10 ==
  note: Configured signal information
  note: Memory address currently being configured
  PID : Inport
  Offset : Inport  Port=2
  ResetDAQ : Inport  Port=3
  Memory_Address : Inport  Port=4
  Signal_Info : Inport  Port=5
  Bus Creator : BusCreator  Inputs=6
  Bus Selector1 : BusSelector  OutputSignals=Signal_Address,Signal_Type,Signal_Conversion
  Detect Rise Positive : simulink/Logic and Bit Operations/Detect Rise Positive  vinit=0  InputProcessing=Inherited  OutDataTypeStr=uint8
  Latch w Update : Subsystem
  Latch w Update1 : Subsystem
  RS Flop-Flop Rp : Subsystem
      mask help: RS flip-flop with priority on R
  Relational Operator2 : RelationalOperator  Operator===  OutDataTypeStr=boolean  RndMeth=Nearest
  Reset Logic : Subsystem
  Terminator : Terminator
  Signal_Data_Updated : Outport
  wires:
  [PID] -> Reset Logic/1(CurrentPID)
  ResetDAQ/1 -> Reset Logic/2(ResetDAQ)
  Reset Logic/1(Reset) -> RS Flop-Flop Rp/1(Rp)
  Bus Selector1/1 -> Relational Operator2/2, Bus Creator/4  "<Signal_Address>"
  Bus Selector1/2 -> Bus Creator/5  "<Signal_Type>"
  Relational Operator2/1 -> RS Flop-Flop Rp/2(S), Detect Rise Positive/1  "F_Signal_Defined"
  Memory_Address/1 -> Relational Operator2/1
  Signal_Info/1 -> Bus Selector1/1
  Bus Creator/1 -> Signal_Data_Updated/1
  Latch w Update/1(Latched) -> [PID], Bus Creator/1  "PID"
  Latch w Update1/1(Latched) -> Bus Creator/2  "Offset"
  Offset/1 -> Latch w Update1/2(In)
  PID/1 -> Latch w Update/2(In)
  Bus Selector1/3 -> Bus Creator/6  "<Signal_Conversion>"
  Detect Rise Positive/1 -> Latch w Update/1(f_update), Latch w Update1/1(f_update)
  RS Flop-Flop Rp/1(Q) -> Bus Creator/3  "F_Defined"
  RS Flop-Flop Rp/2(!Q) -> Terminator/1

== system EmE_MBD_Blockset/User-Defined Functions/Snoop/CCP_ETC_SS1/Signal Data Pairing/Update Signal11 ==
  note: Configured signal information
  note: Memory address currently being configured
  PID : Inport
  Offset : Inport  Port=2
  ResetDAQ : Inport  Port=3
  Memory_Address : Inport  Port=4
  Signal_Info : Inport  Port=5
  Bus Creator : BusCreator  Inputs=6
  Bus Selector1 : BusSelector  OutputSignals=Signal_Address,Signal_Type,Signal_Conversion
  Detect Rise Positive : simulink/Logic and Bit Operations/Detect Rise Positive  vinit=0  InputProcessing=Inherited  OutDataTypeStr=uint8
  Latch w Update : Subsystem
  Latch w Update1 : Subsystem
  RS Flop-Flop Rp : Subsystem
      mask help: RS flip-flop with priority on R
  Relational Operator2 : RelationalOperator  Operator===  OutDataTypeStr=boolean  RndMeth=Nearest
  Reset Logic : Subsystem
  Terminator : Terminator
  Signal_Data_Updated : Outport
  wires:
  [PID] -> Reset Logic/1(CurrentPID)
  ResetDAQ/1 -> Reset Logic/2(ResetDAQ)
  Reset Logic/1(Reset) -> RS Flop-Flop Rp/1(Rp)
  Bus Selector1/1 -> Relational Operator2/2, Bus Creator/4  "<Signal_Address>"
  Bus Selector1/2 -> Bus Creator/5  "<Signal_Type>"
  Relational Operator2/1 -> Detect Rise Positive/1, RS Flop-Flop Rp/2(S)  "F_Signal_Defined"
  Memory_Address/1 -> Relational Operator2/1
  Signal_Info/1 -> Bus Selector1/1
  Bus Creator/1 -> Signal_Data_Updated/1
  Latch w Update/1(Latched) -> [PID], Bus Creator/1  "PID"
  Latch w Update1/1(Latched) -> Bus Creator/2  "Offset"
  Offset/1 -> Latch w Update1/2(In)
  PID/1 -> Latch w Update/2(In)
  Bus Selector1/3 -> Bus Creator/6  "<Signal_Conversion>"
  Detect Rise Positive/1 -> Latch w Update/1(f_update), Latch w Update1/1(f_update)
  RS Flop-Flop Rp/1(Q) -> Bus Creator/3  "F_Defined"
  RS Flop-Flop Rp/2(!Q) -> Terminator/1

== system EmE_MBD_Blockset/User-Defined Functions/Snoop/CCP_ETC_SS1/Signal Data Pairing/Update Signal12 ==
  note: Configured signal information
  note: Memory address currently being configured
  PID : Inport
  Offset : Inport  Port=2
  ResetDAQ : Inport  Port=3
  Memory_Address : Inport  Port=4
  Signal_Info : Inport  Port=5
  Bus Creator : BusCreator  Inputs=6
  Bus Selector1 : BusSelector  OutputSignals=Signal_Address,Signal_Type,Signal_Conversion
  Detect Rise Positive : simulink/Logic and Bit Operations/Detect Rise Positive  vinit=0  InputProcessing=Inherited  OutDataTypeStr=uint8
  Latch w Update : Subsystem
  Latch w Update1 : Subsystem
  RS Flop-Flop Rp : Subsystem
      mask help: RS flip-flop with priority on R
  Relational Operator2 : RelationalOperator  Operator===  OutDataTypeStr=boolean  RndMeth=Nearest
  Reset Logic : Subsystem
  Terminator : Terminator
  Signal_Data_Updated : Outport
  wires:
  [PID] -> Reset Logic/1(CurrentPID)
  ResetDAQ/1 -> Reset Logic/2(ResetDAQ)
  Reset Logic/1(Reset) -> RS Flop-Flop Rp/1(Rp)
  Bus Selector1/1 -> Relational Operator2/2, Bus Creator/4  "<Signal_Address>"
  Bus Selector1/2 -> Bus Creator/5  "<Signal_Type>"
  Relational Operator2/1 -> Detect Rise Positive/1, RS Flop-Flop Rp/2(S)  "F_Signal_Defined"
  Memory_Address/1 -> Relational Operator2/1
  Signal_Info/1 -> Bus Selector1/1
  Bus Creator/1 -> Signal_Data_Updated/1
  Latch w Update/1(Latched) -> [PID], Bus Creator/1  "PID"
  Latch w Update1/1(Latched) -> Bus Creator/2  "Offset"
  Offset/1 -> Latch w Update1/2(In)
  PID/1 -> Latch w Update/2(In)
  Bus Selector1/3 -> Bus Creator/6  "<Signal_Conversion>"
  Detect Rise Positive/1 -> Latch w Update/1(f_update), Latch w Update1/1(f_update)
  RS Flop-Flop Rp/1(Q) -> Bus Creator/3  "F_Defined"
  RS Flop-Flop Rp/2(!Q) -> Terminator/1

== system EmE_MBD_Blockset/User-Defined Functions/Snoop/CCP_ETC_SS1/Signal Data Pairing/Update Signal2 ==
  note: Configured signal information
  note: Memory address currently being configured
  PID : Inport
  Offset : Inport  Port=2
  ResetDAQ : Inport  Port=3
  Memory_Address : Inport  Port=4
  Signal_Info : Inport  Port=5
  Bus Creator : BusCreator  Inputs=6
  Bus Selector1 : BusSelector  OutputSignals=Signal_Address,Signal_Type,Signal_Conversion
  Detect Rise Positive : simulink/Logic and Bit Operations/Detect Rise Positive  vinit=0  InputProcessing=Inherited  OutDataTypeStr=uint8
  Latch w Update : Subsystem
  Latch w Update1 : Subsystem
  RS Flop-Flop Rp : Subsystem
      mask help: RS flip-flop with priority on R
  Relational Operator2 : RelationalOperator  Operator===  OutDataTypeStr=boolean  RndMeth=Nearest
  Reset Logic : Subsystem
  Terminator : Terminator
  Signal_Data_Updated : Outport
  wires:
  [PID] -> Reset Logic/1(CurrentPID)
  ResetDAQ/1 -> Reset Logic/2(ResetDAQ)
  Reset Logic/1(Reset) -> RS Flop-Flop Rp/1(Rp)
  Bus Selector1/1 -> Relational Operator2/2, Bus Creator/4  "<Signal_Address>"
  Bus Selector1/2 -> Bus Creator/5  "<Signal_Type>"
  Relational Operator2/1 -> Detect Rise Positive/1, RS Flop-Flop Rp/2(S)  "F_Signal_Defined"
  Memory_Address/1 -> Relational Operator2/1
  Signal_Info/1 -> Bus Selector1/1
  Bus Creator/1 -> Signal_Data_Updated/1
  Latch w Update/1(Latched) -> [PID], Bus Creator/1  "PID"
  Latch w Update1/1(Latched) -> Bus Creator/2  "Offset"
  Offset/1 -> Latch w Update1/2(In)
  PID/1 -> Latch w Update/2(In)
  Bus Selector1/3 -> Bus Creator/6  "<Signal_Conversion>"
  Detect Rise Positive/1 -> Latch w Update/1(f_update), Latch w Update1/1(f_update)
  RS Flop-Flop Rp/1(Q) -> Bus Creator/3  "F_Defined"
  RS Flop-Flop Rp/2(!Q) -> Terminator/1

== system EmE_MBD_Blockset/User-Defined Functions/Snoop/CCP_ETC_SS1/Signal Data Pairing/Update Signal3 ==
  note: Configured signal information
  note: Memory address currently being configured
  PID : Inport
  Offset : Inport  Port=2
  ResetDAQ : Inport  Port=3
  Memory_Address : Inport  Port=4
  Signal_Info : Inport  Port=5
  Bus Creator : BusCreator  Inputs=6
  Bus Selector1 : BusSelector  OutputSignals=Signal_Address,Signal_Type,Signal_Conversion
  Detect Rise Positive : simulink/Logic and Bit Operations/Detect Rise Positive  vinit=0  InputProcessing=Inherited  OutDataTypeStr=uint8
  Latch w Update : Subsystem
  Latch w Update1 : Subsystem
  RS Flop-Flop Rp : Subsystem
      mask help: RS flip-flop with priority on R
  Relational Operator2 : RelationalOperator  Operator===  OutDataTypeStr=boolean  RndMeth=Nearest
  Reset Logic : Subsystem
  Terminator : Terminator
  Signal_Data_Updated : Outport
  wires:
  [PID] -> Reset Logic/1(CurrentPID)
  ResetDAQ/1 -> Reset Logic/2(ResetDAQ)
  Reset Logic/1(Reset) -> RS Flop-Flop Rp/1(Rp)
  Bus Selector1/1 -> Relational Operator2/2, Bus Creator/4  "<Signal_Address>"
  Bus Selector1/2 -> Bus Creator/5  "<Signal_Type>"
  Relational Operator2/1 -> Detect Rise Positive/1, RS Flop-Flop Rp/2(S)  "F_Signal_Defined"
  Memory_Address/1 -> Relational Operator2/1
  Signal_Info/1 -> Bus Selector1/1
  Bus Creator/1 -> Signal_Data_Updated/1
  Latch w Update/1(Latched) -> [PID], Bus Creator/1  "PID"
  Latch w Update1/1(Latched) -> Bus Creator/2  "Offset"
  Offset/1 -> Latch w Update1/2(In)
  PID/1 -> Latch w Update/2(In)
  Bus Selector1/3 -> Bus Creator/6  "<Signal_Conversion>"
  Detect Rise Positive/1 -> Latch w Update/1(f_update), Latch w Update1/1(f_update)
  RS Flop-Flop Rp/1(Q) -> Bus Creator/3  "F_Defined"
  RS Flop-Flop Rp/2(!Q) -> Terminator/1
